simulink model "OpenLoopControl"  (R2018a)
settings: Solver=FixedStepDiscrete  StartTime=0.0  StopTime=stopTime  FixedStep=sampleTime  RelTol=1e-3
InitFcn:
  | fs=160e3; %Hz
  | stopTime=0.01;
  | sampleTime=1e-8;
  | deadtime= round(((1/fs)/20)/sampleTime);
  | Vdc=100;
  | Lp=82e-6;
  | Cp=1/ (Lp*4*pi*pi*150e3*150e3);
  | Ls=66e-6;
  | Cs=1/ (Ls*4*pi*pi*150e3*150e3);
  | Rp=0.3;
  | Rs=0.2;
  | RLOAD=20
  | k=0.2;
  | M=sqrt(Lp*Ls)*k;
  | Cout=1e-6; %F
libraries: powerlib x20
settings Model: Creator=enes_  LastModifiedBy=enes_

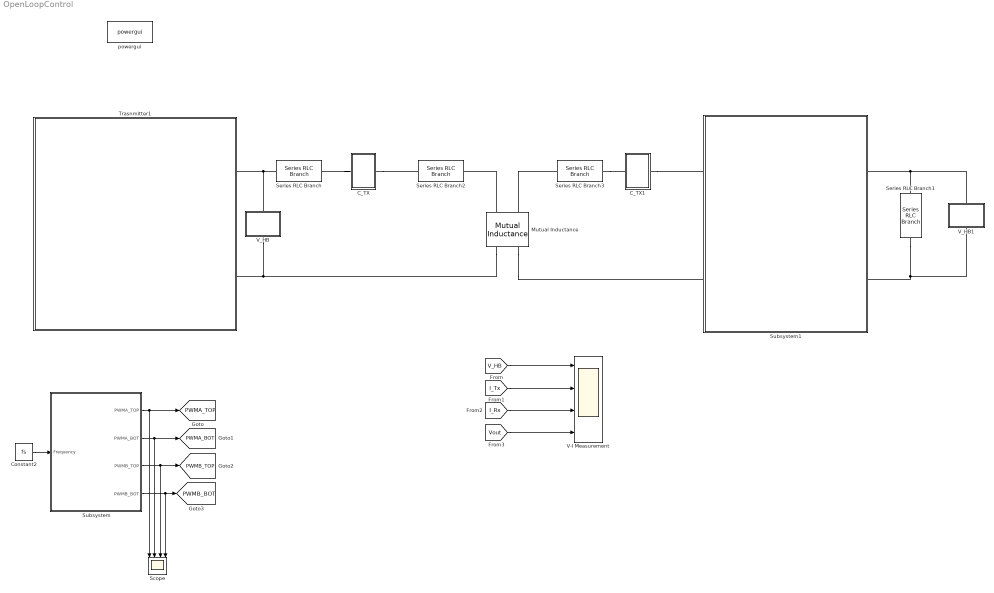
== system OpenLoopControl ==
  C_TX : Subsystem
  C_TX1 : Subsystem
  Constant2 : Constant  Value=fs
  Mutual Inductance : powerlib/Elements/Mutual Inductance  LConnTagsString=a|b  RConnTagsString=A|B  TypeOfMutual=Generalized mutual inductance  NumberOfWindings=2  SelfImpedance1=[1.1 1.1e-03]  SelfImpedance2=[ 1.1 1.1e-03]  ThreeWindings=on  SelfImpedance3=[ 1.1 1.1e-03]  MutualImpedance=[1.0 1.0e-03]  InductanceMatrix=[Lp M ; M Ls]  ResistanceMatrix=[Rp 0; 0 Rs ]  Measurements=None
      settings: AttributesFormatString=\n  SourceProductName=Simscape Power Systems  SourceProductBaseCode=PS
  Scope : Scope  NumInputPorts=4
  Series RLC Branch : powerlib/Elements/Series RLC Branch  LConnTagsString=__new0  RConnTagsString=__new0  BranchType=R  Resistance=Rp  Inductance=Lp  SetiL0=off  InitialCurrent=0  Capacitance=Cp  Setx0=off  InitialVoltage=0  Measurements=None
  Series RLC Branch1 : powerlib/Elements/Series RLC Branch  LConnTagsString=__new0  RConnTagsString=__new0  BranchType=R  Resistance=RLOAD  Inductance=Lp  SetiL0=off  InitialCurrent=0  Capacitance=Cp  Setx0=off  InitialVoltage=0  Measurements=None
  Series RLC Branch2 : powerlib/Elements/Series RLC Branch  LConnTagsString=__new0  RConnTagsString=__new0  BranchType=C  Resistance=Rp  Inductance=Lp  SetiL0=off  InitialCurrent=0  Capacitance=Cp  Setx0=off  InitialVoltage=0  Measurements=None
  Series RLC Branch3 : powerlib/Elements/Series RLC Branch  LConnTagsString=__new0  RConnTagsString=__new0  BranchType=C  Resistance=Rp  Inductance=Lp  SetiL0=off  InitialCurrent=0  Capacitance=Cs  Setx0=off  InitialVoltage=0  Measurements=None
  Subsystem : Subsystem
  Subsystem1 : Subsystem
  Trasnmitter1 : Subsystem
  V-I Measurement : Scope  NumInputPorts=4
  V_HB : Subsystem
  V_HB1 : Subsystem
  powergui : powerlib/powergui  Priority=1  SimulationMode=Discrete  SampleTime=sampleTime  frequency=60  Iterations=50  frequencyindice=0  Pbase=100e6  ErrMax=1e-4  UnitsV=kV  UnitsW=MW  buscounter=0  FunctionMessages=off  echomessages=off  EnableUseOfTLC=off  CurrentSourceSwitches=off  DisableSnubberDevices=off  DisableRonSwitches=off  DisableVfSwitches=off  DisplayEquations=off  SolverType=Tustin/Backward Euler (TBE)  Interpol=off  ExternalGateDelay=off  methode=off  Ts=100  x0status=blocks  SPID=on  SwTol=0  HookPort=off  RestoreLinks=warning  ResistiveCurrentMeasurement=off  Frange=[0:2:500]  Ylog=off  Xlog=on  ShowGrid=off  save=off  variable=ZData  structure=0  ZoomFFT=off  StartTime=0.0  cycles=1  DisplayStyle=1  fundamental=60  FreqAxis=off  MaxFrequency=1000  frequencyindicesteady=1  RmsSteady=1  display=off
  tag scope: PWMA_BOT=global, PWMA_TOP=global, PWMB_BOT=global, PWMB_TOP=global
  wires:
  Constant2/1 -> Subsystem/1(Frequency)
  Subsystem/2(PWMA_BOT) -> [PWMA_BOT], Scope/2
  Subsystem/3(PWMB_TOP) -> [PWMB_TOP], Scope/3
  Subsystem/4(PWMB_BOT) -> [PWMB_BOT], Scope/4
  Subsystem/1(PWMA_TOP) -> [PWMA_TOP], Scope/1
  [V_HB] -> V-I Measurement/1
  [I_Tx] -> V-I Measurement/2
  [I_Rx] -> V-I Measurement/3
  [Vout] -> V-I Measurement/4
  connections:
  Series RLC Branch/LConn1 -- Trasnmitter1/LConn1 -- V_HB/RConn1
  V_HB/LConn1 -- Mutual Inductance/RConn1 -- Trasnmitter1/LConn2
  C_TX/LConn1 -- Series RLC Branch/RConn1
  C_TX/RConn1 -- Series RLC Branch2/LConn1
  Mutual Inductance/LConn1 -- Series RLC Branch2/RConn1
  Mutual Inductance/LConn2 -- Series RLC Branch3/LConn1
  Series RLC Branch3/RConn1 -- C_TX1/LConn1
  V_HB1/RConn1 -- Series RLC Branch1/LConn1 -- Subsystem1/RConn1
  Series RLC Branch1/RConn1 -- V_HB1/LConn1 -- Subsystem1/RConn2
  C_TX1/RConn1 -- Subsystem1/LConn1
  Mutual Inductance/RConn2 -- Subsystem1/LConn2

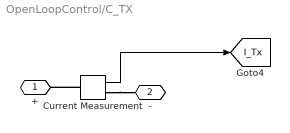
== system OpenLoopControl/C_TX ==
  Current Measurement : powerlib/Measurements/Current Measurement  PhasorSimulation=off  OutputType=Complex  PSBequivalent=0
  + : PMIOPort  Side=Left
  - : PMIOPort  Port=2  Side=Right
  tag scope: I_Tx=global
  wires:
  Current Measurement/1 -> [I_Tx]
  connections:
  Current Measurement/RConn1 -- -/RConn1
  Current Measurement/LConn1 -- +/RConn1

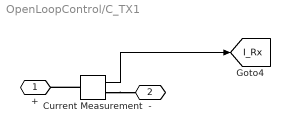
== system OpenLoopControl/C_TX1 ==
  Current Measurement : powerlib/Measurements/Current Measurement  PhasorSimulation=off  OutputType=Complex  PSBequivalent=0
  + : PMIOPort  Side=Left
  - : PMIOPort  Port=2  Side=Right
  tag scope: I_Rx=global
  wires:
  Current Measurement/1 -> [I_Rx]
  connections:
  Current Measurement/RConn1 -- -/RConn1
  Current Measurement/LConn1 -- +/RConn1

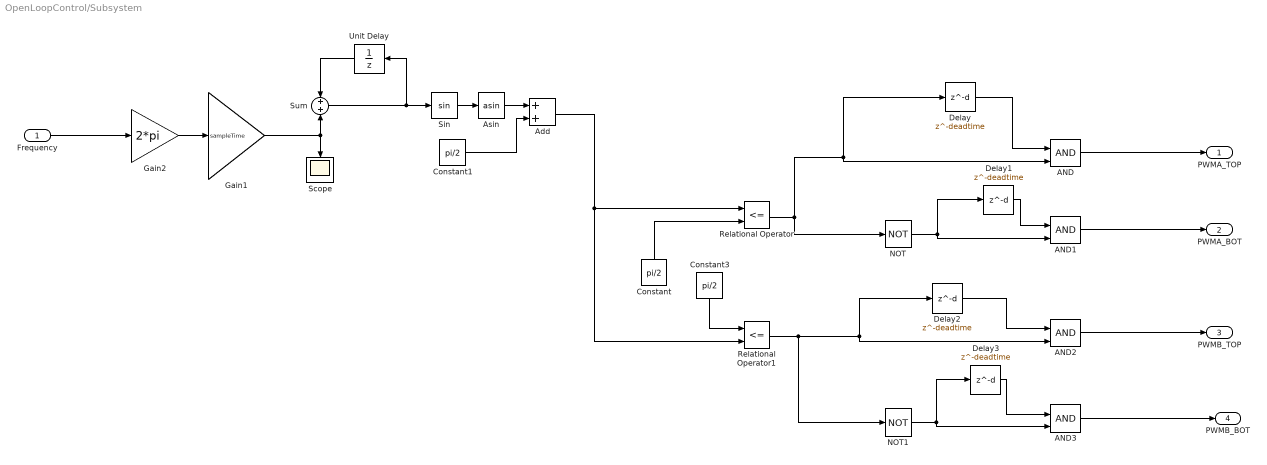
== system OpenLoopControl/Subsystem ==
  Frequency : Inport
  AND{,1..3} (4 alike) : Logic  IconShape=distinctive  AllPortsSameDT=off  OutDataTypeStr=boolean
  Add : Sum
  Asin : Trigonometry  Operator=asin
  Constant : Constant  Value=pi/2
  Constant1 : Constant  Value=pi/2
  Constant3 : Constant  Value=pi/2
  Delay{,1..3} (4 alike) : Delay  DelayLength=deadtime
  Gain1 : Gain  Gain=sampleTime
  Gain2 : Gain  Gain=2*pi
  NOT : Logic  Operator=NOT  IconShape=distinctive  AllPortsSameDT=off  OutDataTypeStr=boolean
  NOT1 : Logic  Operator=NOT  IconShape=distinctive  AllPortsSameDT=off  OutDataTypeStr=boolean
  Relational Operator : RelationalOperator  Operator=<=  OutDataTypeStr=boolean  RndMeth=Simplest
  Relational Operator1 : RelationalOperator  Operator=<=  OutDataTypeStr=boolean  RndMeth=Simplest
  Scope : Scope
  Sin : Trigonometry
  Sum : Sum
  Unit Delay : UnitDelay  SampleTime=-1
  PWMA_TOP : Outport
  PWMA_BOT : Outport  Port=2
  PWMB_TOP : Outport  Port=3
  PWMB_BOT : Outport  Port=4
  wires:
  Gain1/1 -> Sum/2, Scope/1
  AND/1 -> PWMA_TOP/1
  Asin/1 -> Add/1
  Sum/1 -> Sin/1, Unit Delay/1
  Gain2/1 -> Gain1/1
  Unit Delay/1 -> Sum/1
  Constant3/1 -> Relational Operator1/1
  Relational Operator/1 -> NOT/1, Delay/1, AND/2
  AND2/1 -> PWMB_TOP/1
  Frequency/1 -> Gain2/1
  AND3/1 -> PWMB_BOT/1
  NOT1/1 -> Delay3/1, AND3/2
  Add/1 -> Relational Operator1/2, Relational Operator/1
  NOT/1 -> Delay1/1, AND1/2
  AND1/1 -> PWMA_BOT/1
  Delay/1 -> AND/1
  Delay1/1 -> AND1/1
  Relational Operator1/1 -> Delay2/1, AND2/2, NOT1/1
  Delay2/1 -> AND2/1
  Delay3/1 -> AND3/1
  Sin/1 -> Asin/1
  Constant1/1 -> Add/2
  Constant/1 -> Relational Operator/2

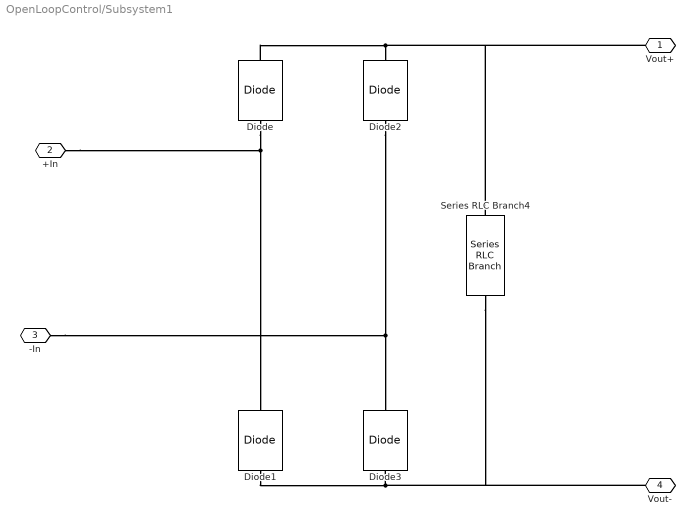
== system OpenLoopControl/Subsystem1 ==
  Diode{,1..3} (4 alike) : powerlib/Power Electronics/Diode  Ron=0.001  Lon=0  Vf=0.8  IC=0  UseSnubber=0  Rs=500  Cs=250e-9  Measurements=off
  Series RLC Branch4 : powerlib/Elements/Series RLC Branch  LConnTagsString=__new0  RConnTagsString=__new0  BranchType=C  Resistance=RLOAD  Inductance=Lp  SetiL0=off  InitialCurrent=0  Capacitance=Cout  Setx0=off  InitialVoltage=0  Measurements=None
  Vout+ : PMIOPort  Side=Right
  +In : PMIOPort  Port=2  Side=Left
  -In : PMIOPort  Port=3  Side=Left
  Vout- : PMIOPort  Port=4  Side=Right
  connections:
  Diode/LConn1 -- +In/RConn1 -- Diode1/RConn1
  Diode/RConn1 -- Vout+/RConn1 -- Series RLC Branch4/LConn1 -- Diode2/RConn1
  Diode2/LConn1 -- Diode3/RConn1 -- -In/RConn1
  Diode1/LConn1 -- Vout-/RConn1 -- Series RLC Branch4/RConn1 -- Diode3/LConn1

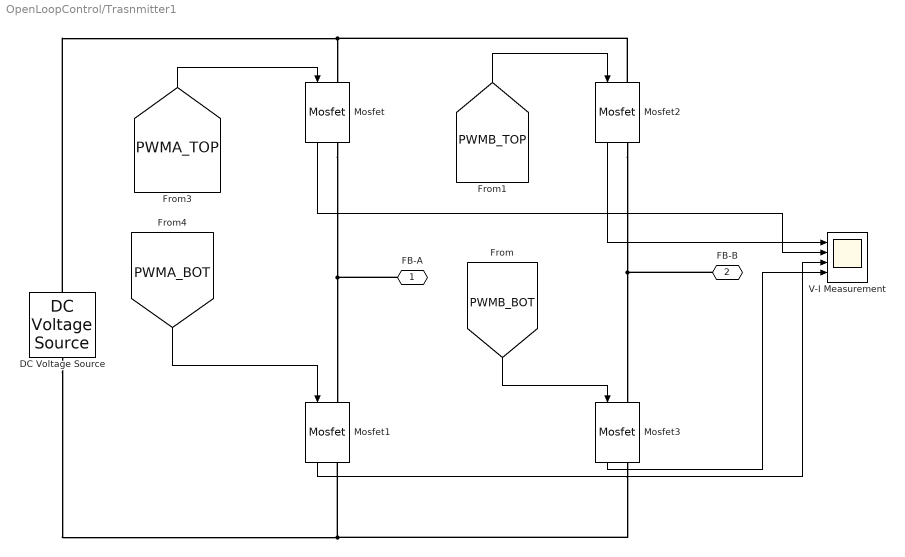
== system OpenLoopControl/Trasnmitter1 ==
  DC Voltage Source : powerlib/Electrical Sources/DC Voltage Source  Amplitude=Vdc  Measurements=None
  Mosfet{,1..3} (4 alike) : powerlib/Power Electronics/Mosfet  Ron=0.1  Lon=0  Rd=0.01  Vfd=0  IC=0  Rs=1e5  Cs=inf  Measurements=on
  V-I Measurement : Scope  NumInputPorts=4
  FB-A : PMIOPort  Side=Left
  FB-B : PMIOPort  Port=2  Side=Left
  wires:
  [PWMA_TOP] -> Mosfet/1
  [PWMB_BOT] -> Mosfet3/1
  [PWMA_BOT] -> Mosfet1/1
  [PWMB_TOP] -> Mosfet2/1
  Mosfet2/1 -> V-I Measurement/1
  Mosfet/1 -> V-I Measurement/2
  Mosfet1/1 -> V-I Measurement/3
  Mosfet3/1 -> V-I Measurement/4
  connections:
  Mosfet2/RConn1 -- FB-B/RConn1 -- Mosfet3/LConn1
  Mosfet/RConn1 -- FB-A/RConn1 -- Mosfet1/LConn1
  DC Voltage Source/RConn1 -- Mosfet2/LConn1 -- Mosfet/LConn1
  DC Voltage Source/LConn1 -- Mosfet3/RConn1 -- Mosfet1/RConn1

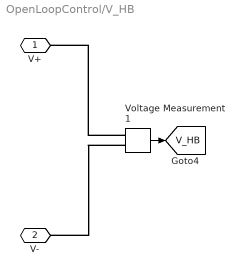
== system OpenLoopControl/V_HB ==
  Voltage Measurement1 : powerlib/Measurements/Voltage Measurement  PhasorSimulation=off  OutputType=Complex  PSBequivalent=0
  V+ : PMIOPort  Side=Right
  V- : PMIOPort  Port=2  Side=Left
  tag scope: V_HB=global
  wires:
  Voltage Measurement1/1 -> [V_HB]
  connections:
  Voltage Measurement1/LConn1 -- V+/RConn1
  Voltage Measurement1/LConn2 -- V-/RConn1

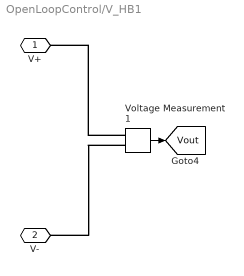
== system OpenLoopControl/V_HB1 ==
  Voltage Measurement1 : powerlib/Measurements/Voltage Measurement  PhasorSimulation=off  OutputType=Complex  PSBequivalent=0
  V+ : PMIOPort  Side=Right
  V- : PMIOPort  Port=2  Side=Left
  tag scope: Vout=global
  wires:
  Voltage Measurement1/1 -> [Vout]
  connections:
  Voltage Measurement1/LConn1 -- V+/RConn1
  Voltage Measurement1/LConn2 -- V-/RConn1
